simulink model "mdlref_house"  (Simulink 6.0)
settings: Solver=ode3  SolverMode=SingleTasking  StartTime=0.0  StopTime=2*24*60*60  FixedStep=60  RelTol=1e-3  AbsTol=1e-6
undefined symbols (not defined in the file or in its folder): c, M, Req, TinIC
settings Model: Creator=The MathWorks Inc.  LastModifiedBy=batserve  ExtModeAutoUpdateStatusClock=off
settings DataIOCC: ExternalInput=[]  InitialState=[]  LimitDataPoints=off  SaveOutput=off  SaveTime=off
settings OptimizationCC: BlockReduction=off  BooleanDataType=off  InlineParams=on
settings DebuggingCC: CheckExecutionContextPreStartOutputMsg=on  CheckExecutionContextRuntimeOutputMsg=on  SignalResolutionControl=UseLocalSettings  SolverPrmCheckMsg=none  IntegerOverflowMsg=none
settings HardwareCC: TargetUnknown=on
settings ModelReferenceCC: ModelReferenceMinAlgLoopOccurrences=on

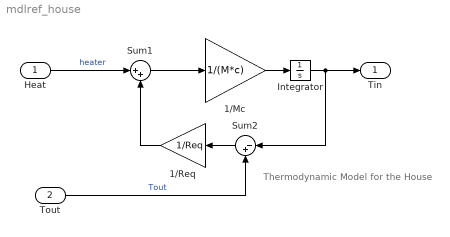
== system mdlref_house ==
  note: Thermodynamic Model
      | for the House
  Heat : Inport  Port=1  PortDimensions=1  SampleTime=0  DataType=double  LatchInput=off
  Tout : Inport  Port=2  PortDimensions=1  SampleTime=0  DataType=double  LatchInput=off
  1/Mc : Gain  Gain=1/(M*c)  SaturateOnIntegerOverflow=on
  1/Req : Gain  Orientation=left  Gain=1/Req  SaturateOnIntegerOverflow=on
  Integrator : Integrator  InitialCondition=TinIC
  Sum1 : Sum  Inputs=|++  SaturateOnIntegerOverflow=on  InputSameDT=on
  Sum2 : Sum  Orientation=left  Inputs=|-+  SaturateOnIntegerOverflow=on  InputSameDT=on
  Tin : Outport  InitialOutput=0
  wires:
  Integrator/1 -> Tin/1, Sum2/1
  1/Mc/1 -> Integrator/1
  1/Req/1 -> Sum1/2
  Sum2/1 -> 1/Req/1
  Sum1/1 -> 1/Mc/1
  Heat/1 -> Sum1/1  "heater"
  Tout/1 -> Sum2/2  "Tout"
